simulink model "P1_Ex2"  (R2021a)
settings: Solver=FixedStepAuto  StartTime=0.0  StopTime=Total_time  RelTol=1e-3
PreLoadFcn:
  | PreLoad_P1_Ex2
StopFcn:
  | post_P1_Ex2
undefined symbols (not defined in the file): Kp, Tg, Ts
libraries: arduinolib x5
settings Model: SimulationMode=external  ExtModeTrigDuration=2  Creator=Eneko Lerma  LastModifiedBy=UPCnet
settings SolverCC: AlgebraicLoopSolver=TrustRegion
settings DataIOCC: ReturnWorkspaceOutputs=off
settings OptimizationCC: EnhancedBackFolding=on  PassReuseOutputArgsAs=Individual arguments  MaxStackSize=64  OptimizeBlockOrder=speed  DifferentSizesBufferReuse=on  OptimizationCustomize=off  EfficientTunableParamExpr=on
settings DebuggingCC: ParameterPrecisionLossMsg=none  ParameterTunabilityLossMsg=error  SFMachineParentedDataDiag=warning  ArithmeticOperatorsInVariantConditions=warning
settings HardwareCC: ProdBitPerPointer=32  ProdBitPerSizeT=32  ProdBitPerPtrDiffT=32  ProdLargestAtomicInteger=Long  ProdLargestAtomicFloat=Double  ProdWordSize=32  ProdHWDeviceType=ARM Compatible->ARM Cortex
settings SFSimCC: SimUseLocalCustomCode=off  MATLABDynamicMemAlloc=off  CustomCodeUndefinedFunction=UseInterfaceOnly
settings RTWCC: SystemTargetFile=ert.tlc  HardwareBoard=Arduino Due  TemplateMakefile=ert_default_tmf  GenerateReport=on  RTWUseLocalCustomCode=off  Toolchain=Arduino ARM  BuildConfiguration=Faster Runs  IncludeHyperlinkInReport=on  LaunchReport=on  GenerateTraceInfo=on  GenerateTraceReport=on  GenerateTraceReportSl=on  GenerateTraceReportSf=on  GenerateTraceReportEml=on
settings RTWCC: CustomTerminator=|
  | writeDigitalPin((uint8_T)3, 0);
  | writeDigitalPin((uint8_T)5, 0);
settings CodeAppCC: ForceParamTrailComments=on  IgnoreCustomStorageClasses=off  OperatorAnnotations=on  SimulinkDataObjDesc=on  SFDataObjDesc=on  InsertBlockDesc=on
settings ERTTargetCC: SupportContinuousTime=on  SupportVariableSizeSignals=on

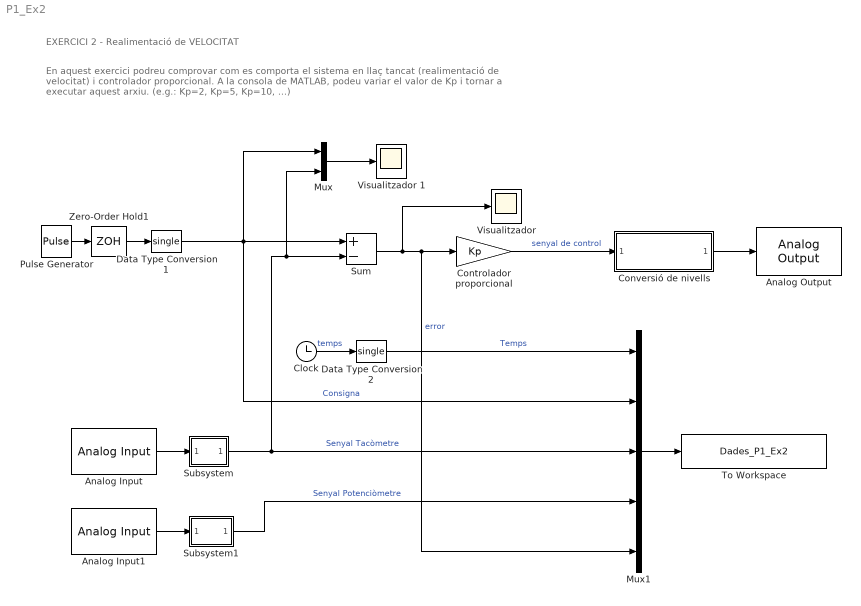
== system P1_Ex2 ==
  note: EXERCICI 2 - Realimentació de VELOCITAT
  note: En aquest exercici podreu comprovar com es comporta el sistema en llaç tancat (realimentació de velocitat)
      | i controlador proporcional. A la consola de MATLAB, podeu variar el valor de Kp i tornar a executar aquest arxiu.
      | (e.g.: Kp=2, Kp=5, Kp=10, ...)
  Analog Input : arduinolib/Analog Input  pinNumber=0  ReadResultsOnly=off  ConversionTriggerSource=Software  ExternalTriggerType=uint32(0)  OutputDataType=uint16  EnableConversionCompleteNotify=off  EnableOuputStatus=off  SampleTime=Tg  blockPlatform=arduino
  Analog Input1 : arduinolib/Analog Input  pinNumber=1  ReadResultsOnly=off  ConversionTriggerSource=Software  ExternalTriggerType=uint32(0)  OutputDataType=uint16  EnableConversionCompleteNotify=off  EnableOuputStatus=off  SampleTime=Tg  blockPlatform=arduino
  Analog Output : arduinolib/Analog Output  DACpin=DAC1  blockPlatform=arduino
      settings: SourceProductBaseCode=ARDUINO
  Clock : Clock
  Controlador proporcional : Gain  Gain=Kp
  Conversió de nivells : Subsystem
  Data Type Conversion1 : DataTypeConversion  OutDataTypeStr=single
  Data Type Conversion2 : DataTypeConversion  OutDataTypeStr=single
  Mux : Mux  Inputs=2
  Mux1 : Mux  Inputs=5
  Pulse Generator : DiscretePulseGenerator  PulseType=Time based  Amplitude=2  Period=5  PulseWidth=50  SampleTime=0.005
  Subsystem : Subsystem
  Subsystem1 : Subsystem
  Sum : Sum  Inputs=+-
  To Workspace : ToWorkspace  VariableName=Dades_P1_Ex2  SampleTime=-1
  Visualitzador : Scope
  Visualitzador 1 : Scope
  Zero-Order Hold1 : ZeroOrderHold  SampleTime=Ts
  wires:
  Controlador proporcional/1 -> Conversió de nivells/1("  ")  "senyal de control"
  Conversió de nivells/1(" ") -> Analog Output/1
  Data Type Conversion1/1 -> Mux1/2, Sum/1, Mux/1  "Consigna"
  Sum/1 -> Controlador proporcional/1, Mux1/5, Visualitzador/1  "error"
  Zero-Order Hold1/1 -> Data Type Conversion1/1
  Mux1/1 -> To Workspace/1
  Clock/1 -> Data Type Conversion2/1  "temps"
  Pulse Generator/1 -> Zero-Order Hold1/1
  Data Type Conversion2/1 -> Mux1/1  "Temps"
  Mux/1 -> Visualitzador 1/1
  Subsystem/1(Out1) -> Sum/2, Mux/2, Mux1/3  "Senyal Tacòmetre"
  Analog Input/1 -> Subsystem/1(In1)
  Analog Input1/1 -> Subsystem1/1(In1)
  Subsystem1/1(Out1) -> Mux1/4  "Senyal Potenciòmetre"

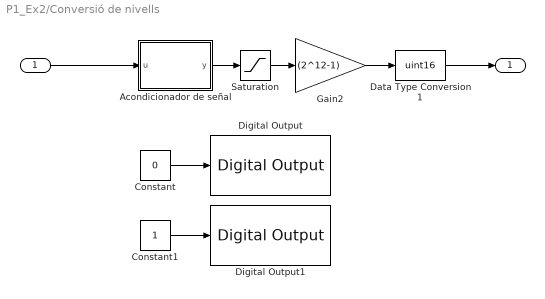
== system P1_Ex2/Conversió de nivells ==
  "  " : Inport  OutDataTypeStr=single
  Acondicionador de señal : MATLAB Function  TreatAsAtomicUnit=on
  Constant : Constant  Value=0
  Constant1 : Constant
  Data Type Conversion1 : DataTypeConversion  OutDataTypeStr=uint16
  Digital Output : arduinolib/Digital Output  pinNumber=3  Direction=output  blockPlatform=arduino
  Digital Output1 : arduinolib/Digital Output  pinNumber=5  Direction=output  blockPlatform=arduino
  Gain2 : Gain  Gain=(2^12-1)  OutDataTypeStr=single
  Saturation : Saturate  UpperLimit=1  LowerLimit=0  OutDataTypeStr=single
  " " : Outport  OutDataTypeStr=uint16  VectorParamsAs1DForOutWhenUnconnected=off
  wires:
  Gain2/1 -> Data Type Conversion1/1
  "  "/1 -> Acondicionador de señal/1(u)
  Acondicionador de señal/1(y) -> Saturation/1
  Data Type Conversion1/1 -> " "/1
  Saturation/1 -> Gain2/1
  Constant/1 -> Digital Output/1
  Constant1/1 -> Digital Output1/1

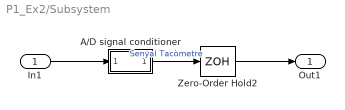
== system P1_Ex2/Subsystem ==
  In1 : Inport
  A/D signal conditioner : Subsystem
  Zero-Order Hold2 : ZeroOrderHold  SampleTime=Ts
  Out1 : Outport  VectorParamsAs1DForOutWhenUnconnected=off
  wires:
  A/D signal conditioner/1(" ") -> Zero-Order Hold2/1  "Senyal Tacòmetre"
  In1/1 -> A/D signal conditioner/1(" ")
  Zero-Order Hold2/1 -> Out1/1

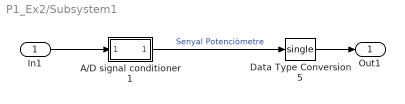
== system P1_Ex2/Subsystem1 ==
  In1 : Inport
  A/D signal conditioner1 : Subsystem
  Data Type Conversion5 : DataTypeConversion  OutDataTypeStr=single
  Out1 : Outport  VectorParamsAs1DForOutWhenUnconnected=off
  wires:
  A/D signal conditioner1/1(" ") -> Data Type Conversion5/1  "Senyal Potenciòmetre"
  Data Type Conversion5/1 -> Out1/1
  In1/1 -> A/D signal conditioner1/1(" ")

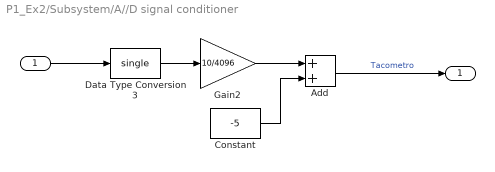
== system P1_Ex2/Subsystem/A//D signal conditioner ==
  " " : Inport
  Add : Sum  AccumDataTypeStr=single
  Constant : Constant  Value=-5  OutDataTypeStr=single
  Data Type Conversion3 : DataTypeConversion  OutDataTypeStr=single
  Gain2 : Gain  Gain=10/4096  OutDataTypeStr=single
  " " : Outport  VectorParamsAs1DForOutWhenUnconnected=off
  wires:
  Data Type Conversion3/1 -> Gain2/1
  Constant/1 -> Add/2
  Gain2/1 -> Add/1
  Add/1 -> " "/1  "Tacometro"
  " "/1 -> Data Type Conversion3/1

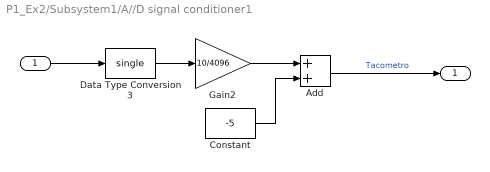
== system P1_Ex2/Subsystem1/A//D signal conditioner1 ==
  " " : Inport
  Add : Sum  AccumDataTypeStr=single
  Constant : Constant  Value=-5  OutDataTypeStr=single  SampleTime=Ts
  Data Type Conversion3 : DataTypeConversion  OutDataTypeStr=single
  Gain2 : Gain  Gain=10/4096  OutDataTypeStr=single
  " " : Outport  VectorParamsAs1DForOutWhenUnconnected=off
  wires:
  Data Type Conversion3/1 -> Gain2/1
  Constant/1 -> Add/2
  Gain2/1 -> Add/1
  Add/1 -> " "/1  "Tacometro"
  " "/1 -> Data Type Conversion3/1

== matlab function P1_Ex2/Conversió de nivells/Acondicionador de señal ==
  data: u input; y output
function y = fcn(u)
y =0.0968*u+0.5058;
